simulink model "six_plus_six_AcmsteeringV09_main_2lflm"  (R2014a)
settings: Solver=FixedStepDiscrete  StartTime=0.0  StopTime=10.0  FixedStep=0.0005  RelTol=1e-3
InitFcn:
  | Veh_Par_wxt
undefined symbols (not defined in the file or in its folder): acc_spdctl, ag_thr, B, bra_em, bra_pre_gz2, bra_pre_gz34, bra_pre_yd, brakepre_dem_data, brakeTrq_dem_data, bratrq_max, ecucoder_acal, eff_tran, ESP_switch, G, guzhang_lf, guzhang_lm, guzhang_lr, guzhang_rf, guzhang_rm, guzhang_rr, kd1, kd2, ki1, ki2, kp1, kp2, L, myFIS, premax, Radius, RC_switch, s_opt_yi, s_opt_zhuan, s_opt_zhuan_add, s_opt_zhuan_table, spd_map_mot, spd_spdctl, speed_thr_park, TCS_switch, tras_ratio, trq_map_mot, trqmax_yd, trqmax_zx, trqmaxneg, v_gain, v_table, v_thr_park, zhidong_bianmazhi, zhidong_down, zhidong_up, zhidong_youmen, zhuanxiang_bianmazhi, zhuanxiang_down, zhuanxiang_up, zhuanxiang_youmen
libraries: simulink x980, ec5744lib x59, fuzblock x2
(part 6 of 25)

== system six_plus_six_AcmsteeringV09_main_2lflm/Data_input/BMS4_2/BMS4 ==
  input : Inport
  Enable : EnablePort
  BMS4_InputVolACC_Ad : Sum
  BMS4_InputVolACC_Convert : DataTypeConversion  OutDataTypeStr=uint32
  BMS4_InputVolACC_F : Gain  Gain=0.1
  BMS4_InputVolACC_L : simulink/Logic and Bit Operations/Bitwise Operator  logicop=AND  UseBitMask=on  BitMask=65535  BitMaskRealWorld=Stored Integer
  BMS4_InputVolACC_O : Constant  Value=0  OutDataTypeStr=single
  BMS4_InputVolACC_S : ArithShift
  BMS4_InputVolACC_Sub : Subsystem
  BMS4_InputVolACC_sat : Saturate  UpperLimit=6553.5  LowerLimit=0
  BMS4_InputVolACCcv : DataTypeConversion
  BMS4_InputVolACCinput2_Ad : Sum
  BMS4_InputVolACCinput2_C : Constant  Value=256
  BMS4_InputVolACCinput2_P : Product
  BMS4_InputVolCHG_Ad : Sum
  BMS4_InputVolCHG_Convert : DataTypeConversion  OutDataTypeStr=uint32
  BMS4_InputVolCHG_F : Gain  Gain=0.1
  BMS4_InputVolCHG_L : simulink/Logic and Bit Operations/Bitwise Operator  logicop=AND  UseBitMask=on  BitMask=65535  BitMaskRealWorld=Stored Integer
  BMS4_InputVolCHG_O : Constant  Value=0  OutDataTypeStr=single
  BMS4_InputVolCHG_S : ArithShift
  BMS4_InputVolCHG_Sub : Subsystem
  BMS4_InputVolCHG_sat : Saturate  UpperLimit=6553.5  LowerLimit=0
  BMS4_InputVolCHGcv : DataTypeConversion
  BMS4_InputVolCHGinput6_Ad : Sum
  BMS4_InputVolCHGinput6_C : Constant  Value=256
  BMS4_InputVolCHGinput6_P : Product
  BMS4_InputVolKEYON_Ad : Sum
  BMS4_InputVolKEYON_Convert : DataTypeConversion  OutDataTypeStr=uint32
  BMS4_InputVolKEYON_F : Gain  Gain=0.1
  BMS4_InputVolKEYON_L : simulink/Logic and Bit Operations/Bitwise Operator  logicop=AND  UseBitMask=on  BitMask=65535  BitMaskRealWorld=Stored Integer
  BMS4_InputVolKEYON_O : Constant  Value=0  OutDataTypeStr=single
  BMS4_InputVolKEYON_S : ArithShift
  BMS4_InputVolKEYON_Sub : Subsystem
  BMS4_InputVolKEYON_sat : Saturate  UpperLimit=6553.5  LowerLimit=0
  BMS4_InputVolKEYONcv : DataTypeConversion
  BMS4_InputVolKEYONinput4_Ad : Sum
  BMS4_InputVolKEYONinput4_C : Constant  Value=256
  BMS4_InputVolKEYONinput4_P : Product
  BMS4_Sys_Status3_Ad : Sum
  BMS4_Sys_Status3_Convert : DataTypeConversion  OutDataTypeStr=uint32
  BMS4_Sys_Status3_F : Gain
  BMS4_Sys_Status3_L : simulink/Logic and Bit Operations/Bitwise Operator  logicop=AND  UseBitMask=on  BitMask=255  BitMaskRealWorld=Stored Integer
  BMS4_Sys_Status3_O : Constant  Value=0  OutDataTypeStr=single
  BMS4_Sys_Status3_S : ArithShift
  BMS4_Sys_Status3_Sub : Subsystem
  BMS4_Sys_Status3_sat : Saturate  UpperLimit=255  LowerLimit=0
  BMS4_Sys_Status3cv : DataTypeConversion
  Demux : Demux  Outputs=8
  BMS4_Sys_Status3_Out : Outport
  BMS4_InputVolKEYON_Out : Outport  Port=2
  BMS4_InputVolCHG_Out : Outport  Port=3
  BMS4_InputVolACC_Out : Outport  Port=4
  wires:
  BMS4_Sys_Status3_F/1 -> BMS4_Sys_Status3_Ad/1
  BMS4_Sys_Status3_O/1 -> BMS4_Sys_Status3_Ad/2
  BMS4_Sys_Status3_Ad/1 -> BMS4_Sys_Status3_sat/1
  BMS4_Sys_Status3_sat/1 -> BMS4_Sys_Status3_Out/1
  Demux/1 -> BMS4_Sys_Status3_Sub/1(In1)
  BMS4_Sys_Status3_Sub/1(Out1) -> BMS4_Sys_Status3_Convert/1
  BMS4_Sys_Status3_Convert/1 -> BMS4_Sys_Status3_L/1
  BMS4_Sys_Status3_L/1 -> BMS4_Sys_Status3_S/1
  BMS4_Sys_Status3_S/1 -> BMS4_Sys_Status3cv/1
  BMS4_Sys_Status3cv/1 -> BMS4_Sys_Status3_F/1
  BMS4_InputVolKEYON_F/1 -> BMS4_InputVolKEYON_Ad/1
  BMS4_InputVolKEYON_O/1 -> BMS4_InputVolKEYON_Ad/2
  BMS4_InputVolKEYON_Ad/1 -> BMS4_InputVolKEYON_sat/1
  BMS4_InputVolKEYON_sat/1 -> BMS4_InputVolKEYON_Out/1
  Demux/4 -> BMS4_InputVolKEYONinput4_P/1
  BMS4_InputVolKEYONinput4_C/1 -> BMS4_InputVolKEYONinput4_P/2
  BMS4_InputVolKEYONinput4_P/1 -> BMS4_InputVolKEYONinput4_Ad/1
  Demux/5 -> BMS4_InputVolKEYONinput4_Ad/2
  BMS4_InputVolKEYONinput4_Ad/1 -> BMS4_InputVolKEYON_Sub/1(In1)
  BMS4_InputVolKEYON_Sub/1(Out1) -> BMS4_InputVolKEYON_Convert/1
  BMS4_InputVolKEYON_Convert/1 -> BMS4_InputVolKEYON_L/1
  BMS4_InputVolKEYON_L/1 -> BMS4_InputVolKEYON_S/1
  BMS4_InputVolKEYON_S/1 -> BMS4_InputVolKEYONcv/1
  BMS4_InputVolKEYONcv/1 -> BMS4_InputVolKEYON_F/1
  BMS4_InputVolCHG_F/1 -> BMS4_InputVolCHG_Ad/1
  BMS4_InputVolCHG_O/1 -> BMS4_InputVolCHG_Ad/2
  BMS4_InputVolCHG_Ad/1 -> BMS4_InputVolCHG_sat/1
  BMS4_InputVolCHG_sat/1 -> BMS4_InputVolCHG_Out/1
  Demux/6 -> BMS4_InputVolCHGinput6_P/1
  BMS4_InputVolCHGinput6_C/1 -> BMS4_InputVolCHGinput6_P/2
  BMS4_InputVolCHGinput6_P/1 -> BMS4_InputVolCHGinput6_Ad/1
  Demux/7 -> BMS4_InputVolCHGinput6_Ad/2
  BMS4_InputVolCHGinput6_Ad/1 -> BMS4_InputVolCHG_Sub/1(In1)
  BMS4_InputVolCHG_Sub/1(Out1) -> BMS4_InputVolCHG_Convert/1
  BMS4_InputVolCHG_Convert/1 -> BMS4_InputVolCHG_L/1
  BMS4_InputVolCHG_L/1 -> BMS4_InputVolCHG_S/1
  BMS4_InputVolCHG_S/1 -> BMS4_InputVolCHGcv/1
  BMS4_InputVolCHGcv/1 -> BMS4_InputVolCHG_F/1
  BMS4_InputVolACC_F/1 -> BMS4_InputVolACC_Ad/1
  BMS4_InputVolACC_O/1 -> BMS4_InputVolACC_Ad/2
  BMS4_InputVolACC_Ad/1 -> BMS4_InputVolACC_sat/1
  BMS4_InputVolACC_sat/1 -> BMS4_InputVolACC_Out/1
  Demux/2 -> BMS4_InputVolACCinput2_P/1
  BMS4_InputVolACCinput2_C/1 -> BMS4_InputVolACCinput2_P/2
  BMS4_InputVolACCinput2_P/1 -> BMS4_InputVolACCinput2_Ad/1
  Demux/3 -> BMS4_InputVolACCinput2_Ad/2
  BMS4_InputVolACCinput2_Ad/1 -> BMS4_InputVolACC_Sub/1(In1)
  BMS4_InputVolACC_Sub/1(Out1) -> BMS4_InputVolACC_Convert/1
  BMS4_InputVolACC_Convert/1 -> BMS4_InputVolACC_L/1
  BMS4_InputVolACC_L/1 -> BMS4_InputVolACC_S/1
  BMS4_InputVolACC_S/1 -> BMS4_InputVolACCcv/1
  BMS4_InputVolACCcv/1 -> BMS4_InputVolACC_F/1
  input/1 -> Demux/1

== system six_plus_six_AcmsteeringV09_main_2lflm/Data_input/BMS5/BMS5 ==
  input : Inport
  Enable : EnablePort
  BMS5_15s_InstanceDisPower_Ad : Sum
  BMS5_15s_InstanceDisPower_Convert : DataTypeConversion  OutDataTypeStr=uint32
  BMS5_15s_InstanceDisPower_F : Gain  Gain=0.01
  BMS5_15s_InstanceDisPower_L : simulink/Logic and Bit Operations/Bitwise Operator  logicop=AND  UseBitMask=on  BitMask=65535  BitMaskRealWorld=Stored Integer
  BMS5_15s_InstanceDisPower_O : Constant  Value=0  OutDataTypeStr=single
  BMS5_15s_InstanceDisPower_S : ArithShift
  BMS5_15s_InstanceDisPower_Sub : Subsystem
  BMS5_15s_InstanceDisPower_sat : Saturate  UpperLimit=655.35  LowerLimit=0
  BMS5_15s_InstanceDisPowercv : DataTypeConversion
  BMS5_15s_InstanceDisPowerinput4_Ad : Sum
  BMS5_15s_InstanceDisPowerinput4_C : Constant  Value=256
  BMS5_15s_InstanceDisPowerinput4_P : Product
  BMS5_ContDischargePower_Ad : Sum
  BMS5_ContDischargePower_Convert : DataTypeConversion  OutDataTypeStr=uint32
  BMS5_ContDischargePower_F : Gain  Gain=0.01
  BMS5_ContDischargePower_L : simulink/Logic and Bit Operations/Bitwise Operator  logicop=AND  UseBitMask=on  BitMask=65535  BitMaskRealWorld=Stored Integer
  BMS5_ContDischargePower_O : Constant  Value=0  OutDataTypeStr=single
  BMS5_ContDischargePower_S : ArithShift
  BMS5_ContDischargePower_Sub : Subsystem
  BMS5_ContDischargePower_sat : Saturate  UpperLimit=655.35  LowerLimit=0
  BMS5_ContDischargePowercv : DataTypeConversion
  BMS5_ContDischargePowerinput2_Ad : Sum
  BMS5_ContDischargePowerinput2_C : Constant  Value=256
  BMS5_ContDischargePowerinput2_P : Product
  BMS5_FailureLevel_Ad : Sum
  BMS5_FailureLevel_Convert : DataTypeConversion  OutDataTypeStr=uint32
  BMS5_FailureLevel_F : Gain
  BMS5_FailureLevel_L : simulink/Logic and Bit Operations/Bitwise Operator  logicop=AND  UseBitMask=on  BitMask=255  BitMaskRealWorld=Stored Integer
  BMS5_FailureLevel_O : Constant  Value=0  OutDataTypeStr=single
  BMS5_FailureLevel_S : ArithShift
  BMS5_FailureLevel_Sub : Subsystem
  BMS5_FailureLevel_sat : Saturate  UpperLimit=255  LowerLimit=0
  BMS5_FailureLevelcv : DataTypeConversion
  BMS5_FeedbackPower_Ad : Sum
  BMS5_FeedbackPower_Convert : DataTypeConversion  OutDataTypeStr=uint32
  BMS5_FeedbackPower_F : Gain  Gain=0.01
  BMS5_FeedbackPower_L : simulink/Logic and Bit Operations/Bitwise Operator  logicop=AND  UseBitMask=on  BitMask=65535  BitMaskRealWorld=Stored Integer
  BMS5_FeedbackPower_O : Constant  Value=0  OutDataTypeStr=single
  BMS5_FeedbackPower_S : ArithShift
  BMS5_FeedbackPower_Sub : Subsystem
  BMS5_FeedbackPower_sat : Saturate  UpperLimit=655.35  LowerLimit=0
  BMS5_FeedbackPowercv : DataTypeConversion
  BMS5_FeedbackPowerinput6_Ad : Sum
  BMS5_FeedbackPowerinput6_C : Constant  Value=256
  BMS5_FeedbackPowerinput6_P : Product
  BMS5_UpDownRequest_Ad : Sum
  BMS5_UpDownRequest_Convert : DataTypeConversion  OutDataTypeStr=uint32
  BMS5_UpDownRequest_F : Gain
  BMS5_UpDownRequest_L : simulink/Logic and Bit Operations/Bitwise Operator  logicop=AND  UseBitMask=on  BitMask=255  BitMaskRealWorld=Stored Integer
  BMS5_UpDownRequest_O : Constant  Value=0  OutDataTypeStr=single
  BMS5_UpDownRequest_S : ArithShift
  BMS5_UpDownRequest_Sub : Subsystem
  BMS5_UpDownRequest_sat : Saturate  UpperLimit=255  LowerLimit=0
  BMS5_UpDownRequestcv : DataTypeConversion
  Demux : Demux  Outputs=8
  BMS5_UpDownRequest_Out : Outport
  BMS5_FeedbackPower_Out : Outport  Port=2
  BMS5_FailureLevel_Out : Outport  Port=3
  BMS5_ContDischargePower_Out : Outport  Port=4
  BMS5_15s_InstanceDisPower_Out : Outport  Port=5
  wires:
  BMS5_UpDownRequest_F/1 -> BMS5_UpDownRequest_Ad/1
  BMS5_UpDownRequest_O/1 -> BMS5_UpDownRequest_Ad/2
  BMS5_UpDownRequest_Ad/1 -> BMS5_UpDownRequest_sat/1
  BMS5_UpDownRequest_sat/1 -> BMS5_UpDownRequest_Out/1
  Demux/8 -> BMS5_UpDownRequest_Sub/1(In1)
  BMS5_UpDownRequest_Sub/1(Out1) -> BMS5_UpDownRequest_Convert/1
  BMS5_UpDownRequest_Convert/1 -> BMS5_UpDownRequest_L/1
  BMS5_UpDownRequest_L/1 -> BMS5_UpDownRequest_S/1
  BMS5_UpDownRequest_S/1 -> BMS5_UpDownRequestcv/1
  BMS5_UpDownRequestcv/1 -> BMS5_UpDownRequest_F/1
  BMS5_FeedbackPower_F/1 -> BMS5_FeedbackPower_Ad/1
  BMS5_FeedbackPower_O/1 -> BMS5_FeedbackPower_Ad/2
  BMS5_FeedbackPower_Ad/1 -> BMS5_FeedbackPower_sat/1
  BMS5_FeedbackPower_sat/1 -> BMS5_FeedbackPower_Out/1
  Demux/6 -> BMS5_FeedbackPowerinput6_P/1
  BMS5_FeedbackPowerinput6_C/1 -> BMS5_FeedbackPowerinput6_P/2
  BMS5_FeedbackPowerinput6_P/1 -> BMS5_FeedbackPowerinput6_Ad/1
  Demux/7 -> BMS5_FeedbackPowerinput6_Ad/2
  BMS5_FeedbackPowerinput6_Ad/1 -> BMS5_FeedbackPower_Sub/1(In1)
  BMS5_FeedbackPower_Sub/1(Out1) -> BMS5_FeedbackPower_Convert/1
  BMS5_FeedbackPower_Convert/1 -> BMS5_FeedbackPower_L/1
  BMS5_FeedbackPower_L/1 -> BMS5_FeedbackPower_S/1
  BMS5_FeedbackPower_S/1 -> BMS5_FeedbackPowercv/1
  BMS5_FeedbackPowercv/1 -> BMS5_FeedbackPower_F/1
  BMS5_FailureLevel_F/1 -> BMS5_FailureLevel_Ad/1
  BMS5_FailureLevel_O/1 -> BMS5_FailureLevel_Ad/2
  BMS5_FailureLevel_Ad/1 -> BMS5_FailureLevel_sat/1
  BMS5_FailureLevel_sat/1 -> BMS5_FailureLevel_Out/1
  Demux/1 -> BMS5_FailureLevel_Sub/1(In1)
  BMS5_FailureLevel_Sub/1(Out1) -> BMS5_FailureLevel_Convert/1
  BMS5_FailureLevel_Convert/1 -> BMS5_FailureLevel_L/1
  BMS5_FailureLevel_L/1 -> BMS5_FailureLevel_S/1
  BMS5_FailureLevel_S/1 -> BMS5_FailureLevelcv/1
  BMS5_FailureLevelcv/1 -> BMS5_FailureLevel_F/1
  BMS5_ContDischargePower_F/1 -> BMS5_ContDischargePower_Ad/1
  BMS5_ContDischargePower_O/1 -> BMS5_ContDischargePower_Ad/2
  BMS5_ContDischargePower_Ad/1 -> BMS5_ContDischargePower_sat/1
  BMS5_ContDischargePower_sat/1 -> BMS5_ContDischargePower_Out/1
  Demux/2 -> BMS5_ContDischargePowerinput2_P/1
  BMS5_ContDischargePowerinput2_C/1 -> BMS5_ContDischargePowerinput2_P/2
  BMS5_ContDischargePowerinput2_P/1 -> BMS5_ContDischargePowerinput2_Ad/1
  Demux/3 -> BMS5_ContDischargePowerinput2_Ad/2
  BMS5_ContDischargePowerinput2_Ad/1 -> BMS5_ContDischargePower_Sub/1(In1)
  BMS5_ContDischargePower_Sub/1(Out1) -> BMS5_ContDischargePower_Convert/1
  BMS5_ContDischargePower_Convert/1 -> BMS5_ContDischargePower_L/1
  BMS5_ContDischargePower_L/1 -> BMS5_ContDischargePower_S/1
  BMS5_ContDischargePower_S/1 -> BMS5_ContDischargePowercv/1
  BMS5_ContDischargePowercv/1 -> BMS5_ContDischargePower_F/1
  BMS5_15s_InstanceDisPower_F/1 -> BMS5_15s_InstanceDisPower_Ad/1
  BMS5_15s_InstanceDisPower_O/1 -> BMS5_15s_InstanceDisPower_Ad/2
  BMS5_15s_InstanceDisPower_Ad/1 -> BMS5_15s_InstanceDisPower_sat/1
  BMS5_15s_InstanceDisPower_sat/1 -> BMS5_15s_InstanceDisPower_Out/1
  Demux/4 -> BMS5_15s_InstanceDisPowerinput4_P/1
  BMS5_15s_InstanceDisPowerinput4_C/1 -> BMS5_15s_InstanceDisPowerinput4_P/2
  BMS5_15s_InstanceDisPowerinput4_P/1 -> BMS5_15s_InstanceDisPowerinput4_Ad/1
  Demux/5 -> BMS5_15s_InstanceDisPowerinput4_Ad/2
  BMS5_15s_InstanceDisPowerinput4_Ad/1 -> BMS5_15s_InstanceDisPower_Sub/1(In1)
  BMS5_15s_InstanceDisPower_Sub/1(Out1) -> BMS5_15s_InstanceDisPower_Convert/1
  BMS5_15s_InstanceDisPower_Convert/1 -> BMS5_15s_InstanceDisPower_L/1
  BMS5_15s_InstanceDisPower_L/1 -> BMS5_15s_InstanceDisPower_S/1
  BMS5_15s_InstanceDisPower_S/1 -> BMS5_15s_InstanceDisPowercv/1
  BMS5_15s_InstanceDisPowercv/1 -> BMS5_15s_InstanceDisPower_F/1
  input/1 -> Demux/1

== system six_plus_six_AcmsteeringV09_main_2lflm/Data_input/BMS5_1/BMS5 ==
  input : Inport
  Enable : EnablePort
  BMS5_15s_InstanceDisPower_Ad : Sum
  BMS5_15s_InstanceDisPower_Convert : DataTypeConversion  OutDataTypeStr=uint32
  BMS5_15s_InstanceDisPower_F : Gain  Gain=0.01
  BMS5_15s_InstanceDisPower_L : simulink/Logic and Bit Operations/Bitwise Operator  logicop=AND  UseBitMask=on  BitMask=65535  BitMaskRealWorld=Stored Integer
  BMS5_15s_InstanceDisPower_O : Constant  Value=0  OutDataTypeStr=single
  BMS5_15s_InstanceDisPower_S : ArithShift
  BMS5_15s_InstanceDisPower_Sub : Subsystem
  BMS5_15s_InstanceDisPower_sat : Saturate  UpperLimit=655.35  LowerLimit=0
  BMS5_15s_InstanceDisPowercv : DataTypeConversion
  BMS5_15s_InstanceDisPowerinput4_Ad : Sum
  BMS5_15s_InstanceDisPowerinput4_C : Constant  Value=256
  BMS5_15s_InstanceDisPowerinput4_P : Product
  BMS5_ContDischargePower_Ad : Sum
  BMS5_ContDischargePower_Convert : DataTypeConversion  OutDataTypeStr=uint32
  BMS5_ContDischargePower_F : Gain  Gain=0.01
  BMS5_ContDischargePower_L : simulink/Logic and Bit Operations/Bitwise Operator  logicop=AND  UseBitMask=on  BitMask=65535  BitMaskRealWorld=Stored Integer
  BMS5_ContDischargePower_O : Constant  Value=0  OutDataTypeStr=single
  BMS5_ContDischargePower_S : ArithShift
  BMS5_ContDischargePower_Sub : Subsystem
  BMS5_ContDischargePower_sat : Saturate  UpperLimit=655.35  LowerLimit=0
  BMS5_ContDischargePowercv : DataTypeConversion
  BMS5_ContDischargePowerinput2_Ad : Sum
  BMS5_ContDischargePowerinput2_C : Constant  Value=256
  BMS5_ContDischargePowerinput2_P : Product
  BMS5_FailureLevel_Ad : Sum
  BMS5_FailureLevel_Convert : DataTypeConversion  OutDataTypeStr=uint32
  BMS5_FailureLevel_F : Gain
  BMS5_FailureLevel_L : simulink/Logic and Bit Operations/Bitwise Operator  logicop=AND  UseBitMask=on  BitMask=255  BitMaskRealWorld=Stored Integer
  BMS5_FailureLevel_O : Constant  Value=0  OutDataTypeStr=single
  BMS5_FailureLevel_S : ArithShift
  BMS5_FailureLevel_Sub : Subsystem
  BMS5_FailureLevel_sat : Saturate  UpperLimit=255  LowerLimit=0
  BMS5_FailureLevelcv : DataTypeConversion
  BMS5_FeedbackPower_Ad : Sum
  BMS5_FeedbackPower_Convert : DataTypeConversion  OutDataTypeStr=uint32
  BMS5_FeedbackPower_F : Gain  Gain=0.01
  BMS5_FeedbackPower_L : simulink/Logic and Bit Operations/Bitwise Operator  logicop=AND  UseBitMask=on  BitMask=65535  BitMaskRealWorld=Stored Integer
  BMS5_FeedbackPower_O : Constant  Value=0  OutDataTypeStr=single
  BMS5_FeedbackPower_S : ArithShift
  BMS5_FeedbackPower_Sub : Subsystem
  BMS5_FeedbackPower_sat : Saturate  UpperLimit=655.35  LowerLimit=0
  BMS5_FeedbackPowercv : DataTypeConversion
  BMS5_FeedbackPowerinput6_Ad : Sum
  BMS5_FeedbackPowerinput6_C : Constant  Value=256
  BMS5_FeedbackPowerinput6_P : Product
  BMS5_UpDownRequest_Ad : Sum
  BMS5_UpDownRequest_Convert : DataTypeConversion  OutDataTypeStr=uint32
  BMS5_UpDownRequest_F : Gain
  BMS5_UpDownRequest_L : simulink/Logic and Bit Operations/Bitwise Operator  logicop=AND  UseBitMask=on  BitMask=255  BitMaskRealWorld=Stored Integer
  BMS5_UpDownRequest_O : Constant  Value=0  OutDataTypeStr=single
  BMS5_UpDownRequest_S : ArithShift
  BMS5_UpDownRequest_Sub : Subsystem
  BMS5_UpDownRequest_sat : Saturate  UpperLimit=255  LowerLimit=0
  BMS5_UpDownRequestcv : DataTypeConversion
  Demux : Demux  Outputs=8
  BMS5_UpDownRequest_Out : Outport
  BMS5_FeedbackPower_Out : Outport  Port=2
  BMS5_FailureLevel_Out : Outport  Port=3
  BMS5_ContDischargePower_Out : Outport  Port=4
  BMS5_15s_InstanceDisPower_Out : Outport  Port=5
  wires:
  BMS5_UpDownRequest_F/1 -> BMS5_UpDownRequest_Ad/1
  BMS5_UpDownRequest_O/1 -> BMS5_UpDownRequest_Ad/2
  BMS5_UpDownRequest_Ad/1 -> BMS5_UpDownRequest_sat/1
  BMS5_UpDownRequest_sat/1 -> BMS5_UpDownRequest_Out/1
  Demux/8 -> BMS5_UpDownRequest_Sub/1(In1)
  BMS5_UpDownRequest_Sub/1(Out1) -> BMS5_UpDownRequest_Convert/1
  BMS5_UpDownRequest_Convert/1 -> BMS5_UpDownRequest_L/1
  BMS5_UpDownRequest_L/1 -> BMS5_UpDownRequest_S/1
  BMS5_UpDownRequest_S/1 -> BMS5_UpDownRequestcv/1
  BMS5_UpDownRequestcv/1 -> BMS5_UpDownRequest_F/1
  BMS5_FeedbackPower_F/1 -> BMS5_FeedbackPower_Ad/1
  BMS5_FeedbackPower_O/1 -> BMS5_FeedbackPower_Ad/2
  BMS5_FeedbackPower_Ad/1 -> BMS5_FeedbackPower_sat/1
  BMS5_FeedbackPower_sat/1 -> BMS5_FeedbackPower_Out/1
  Demux/6 -> BMS5_FeedbackPowerinput6_P/1
  BMS5_FeedbackPowerinput6_C/1 -> BMS5_FeedbackPowerinput6_P/2
  BMS5_FeedbackPowerinput6_P/1 -> BMS5_FeedbackPowerinput6_Ad/1
  Demux/7 -> BMS5_FeedbackPowerinput6_Ad/2
  BMS5_FeedbackPowerinput6_Ad/1 -> BMS5_FeedbackPower_Sub/1(In1)
  BMS5_FeedbackPower_Sub/1(Out1) -> BMS5_FeedbackPower_Convert/1
  BMS5_FeedbackPower_Convert/1 -> BMS5_FeedbackPower_L/1
  BMS5_FeedbackPower_L/1 -> BMS5_FeedbackPower_S/1
  BMS5_FeedbackPower_S/1 -> BMS5_FeedbackPowercv/1
  BMS5_FeedbackPowercv/1 -> BMS5_FeedbackPower_F/1
  BMS5_FailureLevel_F/1 -> BMS5_FailureLevel_Ad/1
  BMS5_FailureLevel_O/1 -> BMS5_FailureLevel_Ad/2
  BMS5_FailureLevel_Ad/1 -> BMS5_FailureLevel_sat/1
  BMS5_FailureLevel_sat/1 -> BMS5_FailureLevel_Out/1
  Demux/1 -> BMS5_FailureLevel_Sub/1(In1)
  BMS5_FailureLevel_Sub/1(Out1) -> BMS5_FailureLevel_Convert/1
  BMS5_FailureLevel_Convert/1 -> BMS5_FailureLevel_L/1
  BMS5_FailureLevel_L/1 -> BMS5_FailureLevel_S/1
  BMS5_FailureLevel_S/1 -> BMS5_FailureLevelcv/1
  BMS5_FailureLevelcv/1 -> BMS5_FailureLevel_F/1
  BMS5_ContDischargePower_F/1 -> BMS5_ContDischargePower_Ad/1
  BMS5_ContDischargePower_O/1 -> BMS5_ContDischargePower_Ad/2
  BMS5_ContDischargePower_Ad/1 -> BMS5_ContDischargePower_sat/1
  BMS5_ContDischargePower_sat/1 -> BMS5_ContDischargePower_Out/1
  Demux/2 -> BMS5_ContDischargePowerinput2_P/1
  BMS5_ContDischargePowerinput2_C/1 -> BMS5_ContDischargePowerinput2_P/2
  BMS5_ContDischargePowerinput2_P/1 -> BMS5_ContDischargePowerinput2_Ad/1
  Demux/3 -> BMS5_ContDischargePowerinput2_Ad/2
  BMS5_ContDischargePowerinput2_Ad/1 -> BMS5_ContDischargePower_Sub/1(In1)
  BMS5_ContDischargePower_Sub/1(Out1) -> BMS5_ContDischargePower_Convert/1
  BMS5_ContDischargePower_Convert/1 -> BMS5_ContDischargePower_L/1
  BMS5_ContDischargePower_L/1 -> BMS5_ContDischargePower_S/1
  BMS5_ContDischargePower_S/1 -> BMS5_ContDischargePowercv/1
  BMS5_ContDischargePowercv/1 -> BMS5_ContDischargePower_F/1
  BMS5_15s_InstanceDisPower_F/1 -> BMS5_15s_InstanceDisPower_Ad/1
  BMS5_15s_InstanceDisPower_O/1 -> BMS5_15s_InstanceDisPower_Ad/2
  BMS5_15s_InstanceDisPower_Ad/1 -> BMS5_15s_InstanceDisPower_sat/1
  BMS5_15s_InstanceDisPower_sat/1 -> BMS5_15s_InstanceDisPower_Out/1
  Demux/4 -> BMS5_15s_InstanceDisPowerinput4_P/1
  BMS5_15s_InstanceDisPowerinput4_C/1 -> BMS5_15s_InstanceDisPowerinput4_P/2
  BMS5_15s_InstanceDisPowerinput4_P/1 -> BMS5_15s_InstanceDisPowerinput4_Ad/1
  Demux/5 -> BMS5_15s_InstanceDisPowerinput4_Ad/2
  BMS5_15s_InstanceDisPowerinput4_Ad/1 -> BMS5_15s_InstanceDisPower_Sub/1(In1)
  BMS5_15s_InstanceDisPower_Sub/1(Out1) -> BMS5_15s_InstanceDisPower_Convert/1
  BMS5_15s_InstanceDisPower_Convert/1 -> BMS5_15s_InstanceDisPower_L/1
  BMS5_15s_InstanceDisPower_L/1 -> BMS5_15s_InstanceDisPower_S/1
  BMS5_15s_InstanceDisPower_S/1 -> BMS5_15s_InstanceDisPowercv/1
  BMS5_15s_InstanceDisPowercv/1 -> BMS5_15s_InstanceDisPower_F/1
  input/1 -> Demux/1

== system six_plus_six_AcmsteeringV09_main_2lflm/Data_input/BMS5_2/BMS5 ==
  input : Inport
  Enable : EnablePort
  BMS5_15s_InstanceDisPower_Ad : Sum
  BMS5_15s_InstanceDisPower_Convert : DataTypeConversion  OutDataTypeStr=uint32
  BMS5_15s_InstanceDisPower_F : Gain  Gain=0.01
  BMS5_15s_InstanceDisPower_L : simulink/Logic and Bit Operations/Bitwise Operator  logicop=AND  UseBitMask=on  BitMask=65535  BitMaskRealWorld=Stored Integer
  BMS5_15s_InstanceDisPower_O : Constant  Value=0  OutDataTypeStr=single
  BMS5_15s_InstanceDisPower_S : ArithShift
  BMS5_15s_InstanceDisPower_Sub : Subsystem
  BMS5_15s_InstanceDisPower_sat : Saturate  UpperLimit=655.35  LowerLimit=0
  BMS5_15s_InstanceDisPowercv : DataTypeConversion
  BMS5_15s_InstanceDisPowerinput4_Ad : Sum
  BMS5_15s_InstanceDisPowerinput4_C : Constant  Value=256
  BMS5_15s_InstanceDisPowerinput4_P : Product
  BMS5_ContDischargePower_Ad : Sum
  BMS5_ContDischargePower_Convert : DataTypeConversion  OutDataTypeStr=uint32
  BMS5_ContDischargePower_F : Gain  Gain=0.01
  BMS5_ContDischargePower_L : simulink/Logic and Bit Operations/Bitwise Operator  logicop=AND  UseBitMask=on  BitMask=65535  BitMaskRealWorld=Stored Integer
  BMS5_ContDischargePower_O : Constant  Value=0  OutDataTypeStr=single
  BMS5_ContDischargePower_S : ArithShift
  BMS5_ContDischargePower_Sub : Subsystem
  BMS5_ContDischargePower_sat : Saturate  UpperLimit=655.35  LowerLimit=0
  BMS5_ContDischargePowercv : DataTypeConversion
  BMS5_ContDischargePowerinput2_Ad : Sum
  BMS5_ContDischargePowerinput2_C : Constant  Value=256
  BMS5_ContDischargePowerinput2_P : Product
  BMS5_FailureLevel_Ad : Sum
  BMS5_FailureLevel_Convert : DataTypeConversion  OutDataTypeStr=uint32
  BMS5_FailureLevel_F : Gain
  BMS5_FailureLevel_L : simulink/Logic and Bit Operations/Bitwise Operator  logicop=AND  UseBitMask=on  BitMask=255  BitMaskRealWorld=Stored Integer
  BMS5_FailureLevel_O : Constant  Value=0  OutDataTypeStr=single
  BMS5_FailureLevel_S : ArithShift
  BMS5_FailureLevel_Sub : Subsystem
  BMS5_FailureLevel_sat : Saturate  UpperLimit=255  LowerLimit=0
  BMS5_FailureLevelcv : DataTypeConversion
  BMS5_FeedbackPower_Ad : Sum
  BMS5_FeedbackPower_Convert : DataTypeConversion  OutDataTypeStr=uint32
  BMS5_FeedbackPower_F : Gain  Gain=0.01
  BMS5_FeedbackPower_L : simulink/Logic and Bit Operations/Bitwise Operator  logicop=AND  UseBitMask=on  BitMask=65535  BitMaskRealWorld=Stored Integer
  BMS5_FeedbackPower_O : Constant  Value=0  OutDataTypeStr=single
  BMS5_FeedbackPower_S : ArithShift
  BMS5_FeedbackPower_Sub : Subsystem
  BMS5_FeedbackPower_sat : Saturate  UpperLimit=655.35  LowerLimit=0
  BMS5_FeedbackPowercv : DataTypeConversion
  BMS5_FeedbackPowerinput6_Ad : Sum
  BMS5_FeedbackPowerinput6_C : Constant  Value=256
  BMS5_FeedbackPowerinput6_P : Product
  BMS5_UpDownRequest_Ad : Sum
  BMS5_UpDownRequest_Convert : DataTypeConversion  OutDataTypeStr=uint32
  BMS5_UpDownRequest_F : Gain
  BMS5_UpDownRequest_L : simulink/Logic and Bit Operations/Bitwise Operator  logicop=AND  UseBitMask=on  BitMask=255  BitMaskRealWorld=Stored Integer
  BMS5_UpDownRequest_O : Constant  Value=0  OutDataTypeStr=single
  BMS5_UpDownRequest_S : ArithShift
  BMS5_UpDownRequest_Sub : Subsystem
  BMS5_UpDownRequest_sat : Saturate  UpperLimit=255  LowerLimit=0
  BMS5_UpDownRequestcv : DataTypeConversion
  Demux : Demux  Outputs=8
  BMS5_UpDownRequest_Out : Outport
  BMS5_FeedbackPower_Out : Outport  Port=2
  BMS5_FailureLevel_Out : Outport  Port=3
  BMS5_ContDischargePower_Out : Outport  Port=4
  BMS5_15s_InstanceDisPower_Out : Outport  Port=5
  wires:
  BMS5_UpDownRequest_F/1 -> BMS5_UpDownRequest_Ad/1
  BMS5_UpDownRequest_O/1 -> BMS5_UpDownRequest_Ad/2
  BMS5_UpDownRequest_Ad/1 -> BMS5_UpDownRequest_sat/1
  BMS5_UpDownRequest_sat/1 -> BMS5_UpDownRequest_Out/1
  Demux/8 -> BMS5_UpDownRequest_Sub/1(In1)
  BMS5_UpDownRequest_Sub/1(Out1) -> BMS5_UpDownRequest_Convert/1
  BMS5_UpDownRequest_Convert/1 -> BMS5_UpDownRequest_L/1
  BMS5_UpDownRequest_L/1 -> BMS5_UpDownRequest_S/1
  BMS5_UpDownRequest_S/1 -> BMS5_UpDownRequestcv/1
  BMS5_UpDownRequestcv/1 -> BMS5_UpDownRequest_F/1
  BMS5_FeedbackPower_F/1 -> BMS5_FeedbackPower_Ad/1
  BMS5_FeedbackPower_O/1 -> BMS5_FeedbackPower_Ad/2
  BMS5_FeedbackPower_Ad/1 -> BMS5_FeedbackPower_sat/1
  BMS5_FeedbackPower_sat/1 -> BMS5_FeedbackPower_Out/1
  Demux/6 -> BMS5_FeedbackPowerinput6_P/1
  BMS5_FeedbackPowerinput6_C/1 -> BMS5_FeedbackPowerinput6_P/2
  BMS5_FeedbackPowerinput6_P/1 -> BMS5_FeedbackPowerinput6_Ad/1
  Demux/7 -> BMS5_FeedbackPowerinput6_Ad/2
  BMS5_FeedbackPowerinput6_Ad/1 -> BMS5_FeedbackPower_Sub/1(In1)
  BMS5_FeedbackPower_Sub/1(Out1) -> BMS5_FeedbackPower_Convert/1
  BMS5_FeedbackPower_Convert/1 -> BMS5_FeedbackPower_L/1
  BMS5_FeedbackPower_L/1 -> BMS5_FeedbackPower_S/1
  BMS5_FeedbackPower_S/1 -> BMS5_FeedbackPowercv/1
  BMS5_FeedbackPowercv/1 -> BMS5_FeedbackPower_F/1
  BMS5_FailureLevel_F/1 -> BMS5_FailureLevel_Ad/1
  BMS5_FailureLevel_O/1 -> BMS5_FailureLevel_Ad/2
  BMS5_FailureLevel_Ad/1 -> BMS5_FailureLevel_sat/1
  BMS5_FailureLevel_sat/1 -> BMS5_FailureLevel_Out/1
  Demux/1 -> BMS5_FailureLevel_Sub/1(In1)
  BMS5_FailureLevel_Sub/1(Out1) -> BMS5_FailureLevel_Convert/1
  BMS5_FailureLevel_Convert/1 -> BMS5_FailureLevel_L/1
  BMS5_FailureLevel_L/1 -> BMS5_FailureLevel_S/1
  BMS5_FailureLevel_S/1 -> BMS5_FailureLevelcv/1
  BMS5_FailureLevelcv/1 -> BMS5_FailureLevel_F/1
  BMS5_ContDischargePower_F/1 -> BMS5_ContDischargePower_Ad/1
  BMS5_ContDischargePower_O/1 -> BMS5_ContDischargePower_Ad/2
  BMS5_ContDischargePower_Ad/1 -> BMS5_ContDischargePower_sat/1
  BMS5_ContDischargePower_sat/1 -> BMS5_ContDischargePower_Out/1
  Demux/2 -> BMS5_ContDischargePowerinput2_P/1
  BMS5_ContDischargePowerinput2_C/1 -> BMS5_ContDischargePowerinput2_P/2
  BMS5_ContDischargePowerinput2_P/1 -> BMS5_ContDischargePowerinput2_Ad/1
  Demux/3 -> BMS5_ContDischargePowerinput2_Ad/2
  BMS5_ContDischargePowerinput2_Ad/1 -> BMS5_ContDischargePower_Sub/1(In1)
  BMS5_ContDischargePower_Sub/1(Out1) -> BMS5_ContDischargePower_Convert/1
  BMS5_ContDischargePower_Convert/1 -> BMS5_ContDischargePower_L/1
  BMS5_ContDischargePower_L/1 -> BMS5_ContDischargePower_S/1
  BMS5_ContDischargePower_S/1 -> BMS5_ContDischargePowercv/1
  BMS5_ContDischargePowercv/1 -> BMS5_ContDischargePower_F/1
  BMS5_15s_InstanceDisPower_F/1 -> BMS5_15s_InstanceDisPower_Ad/1
  BMS5_15s_InstanceDisPower_O/1 -> BMS5_15s_InstanceDisPower_Ad/2
  BMS5_15s_InstanceDisPower_Ad/1 -> BMS5_15s_InstanceDisPower_sat/1
  BMS5_15s_InstanceDisPower_sat/1 -> BMS5_15s_InstanceDisPower_Out/1
  Demux/4 -> BMS5_15s_InstanceDisPowerinput4_P/1
  BMS5_15s_InstanceDisPowerinput4_C/1 -> BMS5_15s_InstanceDisPowerinput4_P/2
  BMS5_15s_InstanceDisPowerinput4_P/1 -> BMS5_15s_InstanceDisPowerinput4_Ad/1
  Demux/5 -> BMS5_15s_InstanceDisPowerinput4_Ad/2
  BMS5_15s_InstanceDisPowerinput4_Ad/1 -> BMS5_15s_InstanceDisPower_Sub/1(In1)
  BMS5_15s_InstanceDisPower_Sub/1(Out1) -> BMS5_15s_InstanceDisPower_Convert/1
  BMS5_15s_InstanceDisPower_Convert/1 -> BMS5_15s_InstanceDisPower_L/1
  BMS5_15s_InstanceDisPower_L/1 -> BMS5_15s_InstanceDisPower_S/1
  BMS5_15s_InstanceDisPower_S/1 -> BMS5_15s_InstanceDisPowercv/1
  BMS5_15s_InstanceDisPowercv/1 -> BMS5_15s_InstanceDisPower_F/1
  input/1 -> Demux/1

== system six_plus_six_AcmsteeringV09_main_2lflm/Data_input/Enabled Subsystem/Subsystem ==
  CANTransmit : ec5744lib/RapidECU_U3/04CANCommunication/CANTransmit  canmodule=1  canbuffer=59  canmessageid=hex2dec('0000')  canmessagetype=Standard(11-bit ID)  datalength=2  sampletime=-1
  Constant2 : Constant  Value=hex2dec('00')  SampleTime=-1
  Constant3 : Constant  Value=hex2dec('01')  SampleTime=-1
  Data Type Conversion3 : DataTypeConversion
  Data Type Conversion8 : DataTypeConversion
  Mux : Mux  Inputs=2
  Terminator2 : Terminator
  wires:
  Mux/1 -> CANTransmit/1
  Constant3/1 -> Data Type Conversion3/1
  CANTransmit/1 -> Terminator2/1
  Data Type Conversion3/1 -> Mux/1
  Data Type Conversion8/1 -> Mux/2
  Constant2/1 -> Data Type Conversion8/1

== system six_plus_six_AcmsteeringV09_main_2lflm/Data_input/MCU0/MCU0 ==
  input : Inport
  Enable : EnablePort
  Demux : Demux  Outputs=8
  MCU0_ControlMode_Ad : Sum
  MCU0_ControlMode_Convert : DataTypeConversion  OutDataTypeStr=uint32
  MCU0_ControlMode_F : Gain
  MCU0_ControlMode_L : simulink/Logic and Bit Operations/Bitwise Operator  logicop=AND  UseBitMask=on  BitMask=4  BitMaskRealWorld=Stored Integer
  MCU0_ControlMode_O : Constant  Value=0  OutDataTypeStr=single
  MCU0_ControlMode_S : ArithShift  BitShiftNumber=2
  MCU0_ControlMode_Sub : Subsystem
  MCU0_ControlMode_sat : Saturate  UpperLimit=1  LowerLimit=0
  MCU0_ControlModecv : DataTypeConversion
  MCU0_EmergShutDown_Ad : Sum
  MCU0_EmergShutDown_Convert : DataTypeConversion  OutDataTypeStr=uint32
  MCU0_EmergShutDown_F : Gain
  MCU0_EmergShutDown_L : simulink/Logic and Bit Operations/Bitwise Operator  logicop=AND  UseBitMask=on  BitMask=128  BitMaskRealWorld=Stored Integer
  MCU0_EmergShutDown_O : Constant  Value=0  OutDataTypeStr=single
  MCU0_EmergShutDown_S : ArithShift  BitShiftNumber=7
  MCU0_EmergShutDown_Sub : Subsystem
  MCU0_EmergShutDown_sat : Saturate  UpperLimit=1  LowerLimit=0
  MCU0_EmergShutDowncv : DataTypeConversion
  MCU0_GearStatus_Ad : Sum
  MCU0_GearStatus_Convert : DataTypeConversion  OutDataTypeStr=uint32
  MCU0_GearStatus_F : Gain
  MCU0_GearStatus_L : simulink/Logic and Bit Operations/Bitwise Operator  logicop=AND  UseBitMask=on  BitMask=24  BitMaskRealWorld=Stored Integer
  MCU0_GearStatus_O : Constant  Value=0  OutDataTypeStr=single
  MCU0_GearStatus_S : ArithShift  BitShiftNumber=3
  MCU0_GearStatus_Sub : Subsystem
  MCU0_GearStatus_sat : Saturate  UpperLimit=3  LowerLimit=0
  MCU0_GearStatuscv : DataTypeConversion
  MCU0_HighVol_Ad : Sum
  MCU0_HighVol_Convert : DataTypeConversion  OutDataTypeStr=uint32
  MCU0_HighVol_F : Gain
  MCU0_HighVol_L : simulink/Logic and Bit Operations/Bitwise Operator  logicop=AND  UseBitMask=on  BitMask=32  BitMaskRealWorld=Stored Integer
  MCU0_HighVol_O : Constant  Value=0  OutDataTypeStr=single
  MCU0_HighVol_S : ArithShift  BitShiftNumber=5
  MCU0_HighVol_Sub : Subsystem
  MCU0_HighVol_sat : Saturate  UpperLimit=1  LowerLimit=0
  MCU0_HighVolcv : DataTypeConversion
  MCU0_LiftCnt_Ad : Sum
  MCU0_LiftCnt_Convert : DataTypeConversion  OutDataTypeStr=uint32
  MCU0_LiftCnt_F : Gain
  MCU0_LiftCnt_L : simulink/Logic and Bit Operations/Bitwise Operator  logicop=AND  UseBitMask=on  BitMask=255  BitMaskRealWorld=Stored Integer
  MCU0_LiftCnt_O : Constant  Value=0  OutDataTypeStr=single
  MCU0_LiftCnt_S : ArithShift
  MCU0_LiftCnt_Sub : Subsystem
  MCU0_LiftCnt_sat : Saturate  UpperLimit=255  LowerLimit=0
  MCU0_LiftCntcv : DataTypeConversion
  MCU0_ShutDowAllow_Ad : Sum
  MCU0_ShutDowAllow_Convert : DataTypeConversion  OutDataTypeStr=uint32
  MCU0_ShutDowAllow_F : Gain
  MCU0_ShutDowAllow_L : simulink/Logic and Bit Operations/Bitwise Operator  logicop=AND  UseBitMask=on  BitMask=64  BitMaskRealWorld=Stored Integer
  MCU0_ShutDowAllow_O : Constant  Value=0  OutDataTypeStr=single
  MCU0_ShutDowAllow_S : ArithShift  BitShiftNumber=6
  MCU0_ShutDowAllow_Sub : Subsystem
  MCU0_ShutDowAllow_sat : Saturate  UpperLimit=1  LowerLimit=0
  MCU0_ShutDowAllowcv : DataTypeConversion
  MCU0_SpeedFdk_Ad : Sum
  MCU0_SpeedFdk_Convert : DataTypeConversion  OutDataTypeStr=uint32
  MCU0_SpeedFdk_F : Gain
  MCU0_SpeedFdk_L : simulink/Logic and Bit Operations/Bitwise Operator  logicop=AND  UseBitMask=on  BitMask=65535  BitMaskRealWorld=Stored Integer
  MCU0_SpeedFdk_O : Constant  Value=-10000  OutDataTypeStr=single
  MCU0_SpeedFdk_S : ArithShift
  MCU0_SpeedFdk_Sub : Subsystem
  MCU0_SpeedFdk_sat : Saturate  UpperLimit=10000  LowerLimit=-10000
  MCU0_SpeedFdkcv : DataTypeConversion
  MCU0_SpeedFdkinput2_Ad : Sum
  MCU0_SpeedFdkinput2_C : Constant  Value=256
  MCU0_SpeedFdkinput2_P : Product
  MCU0_TorqueFdk_Ad : Sum
  MCU0_TorqueFdk_Convert : DataTypeConversion  OutDataTypeStr=uint32
  MCU0_TorqueFdk_F : Gain  Gain=0.1
  MCU0_TorqueFdk_L : simulink/Logic and Bit Operations/Bitwise Operator  logicop=AND  UseBitMask=on  BitMask=65535  BitMaskRealWorld=Stored Integer
  MCU0_TorqueFdk_O : Constant  Value=-1000  OutDataTypeStr=single
  MCU0_TorqueFdk_S : ArithShift
  MCU0_TorqueFdk_Sub : Subsystem
  MCU0_TorqueFdk_sat : Saturate  UpperLimit=1000  LowerLimit=-1000
  MCU0_TorqueFdkcv : DataTypeConversion
  MCU0_TorqueFdkinput4_Ad : Sum
  MCU0_TorqueFdkinput4_C : Constant  Value=256
  MCU0_TorqueFdkinput4_P : Product
  MCU0_TorqueMax_Ad : Sum
  MCU0_TorqueMax_Convert : DataTypeConversion  OutDataTypeStr=uint32
  MCU0_TorqueMax_F : Gain  Gain=0.1
  MCU0_TorqueMax_L : simulink/Logic and Bit Operations/Bitwise Operator  logicop=AND  UseBitMask=on  BitMask=65535  BitMaskRealWorld=Stored Integer
  MCU0_TorqueMax_O : Constant  Value=-1000  OutDataTypeStr=single
  MCU0_TorqueMax_S : ArithShift
  MCU0_TorqueMax_Sub : Subsystem
  MCU0_TorqueMax_sat : Saturate  UpperLimit=1000  LowerLimit=-1000
  MCU0_TorqueMaxcv : DataTypeConversion
  MCU0_TorqueMaxinput6_Ad : Sum
  MCU0_TorqueMaxinput6_C : Constant  Value=256
  MCU0_TorqueMaxinput6_P : Product
  MCU0_WorkStatus_Ad : Sum
  MCU0_WorkStatus_Convert : DataTypeConversion  OutDataTypeStr=uint32
  MCU0_WorkStatus_F : Gain
  MCU0_WorkStatus_L : simulink/Logic and Bit Operations/Bitwise Operator  logicop=AND  UseBitMask=on  BitMask=3  BitMaskRealWorld=Stored Integer
  MCU0_WorkStatus_O : Constant  Value=0  OutDataTypeStr=single
  MCU0_WorkStatus_S : ArithShift
  MCU0_WorkStatus_Sub : Subsystem
  MCU0_WorkStatus_sat : Saturate  UpperLimit=3  LowerLimit=0
  MCU0_WorkStatuscv : DataTypeConversion
  MCU0_TorqueMax_Out : Outport
  MCU0_EmergShutDown_Out : Outport  Port=2
  MCU0_ShutDowAllow_Out : Outport  Port=3
  MCU0_HighVol_Out : Outport  Port=4
  MCU0_LiftCnt_Out : Outport  Port=5
  MCU0_TorqueFdk_Out : Outport  Port=6
  MCU0_SpeedFdk_Out : Outport  Port=7
  MCU0_GearStatus_Out : Outport  Port=8
  MCU0_ControlMode_Out : Outport  Port=9
  MCU0_WorkStatus_Out : Outport  Port=10
  wires:
  MCU0_TorqueMax_F/1 -> MCU0_TorqueMax_Ad/1
  MCU0_TorqueMax_O/1 -> MCU0_TorqueMax_Ad/2
  MCU0_TorqueMax_Ad/1 -> MCU0_TorqueMax_sat/1
  MCU0_TorqueMax_sat/1 -> MCU0_TorqueMax_Out/1
  Demux/6 -> MCU0_TorqueMaxinput6_P/1
  MCU0_TorqueMaxinput6_C/1 -> MCU0_TorqueMaxinput6_P/2
  MCU0_TorqueMaxinput6_P/1 -> MCU0_TorqueMaxinput6_Ad/1
  Demux/7 -> MCU0_TorqueMaxinput6_Ad/2
  MCU0_TorqueMaxinput6_Ad/1 -> MCU0_TorqueMax_Sub/1(In1)
  MCU0_TorqueMax_Sub/1(Out1) -> MCU0_TorqueMax_Convert/1
  MCU0_TorqueMax_Convert/1 -> MCU0_TorqueMax_L/1
  MCU0_TorqueMax_L/1 -> MCU0_TorqueMax_S/1
  MCU0_TorqueMax_S/1 -> MCU0_TorqueMaxcv/1
  MCU0_TorqueMaxcv/1 -> MCU0_TorqueMax_F/1
  MCU0_EmergShutDown_F/1 -> MCU0_EmergShutDown_Ad/1
  MCU0_EmergShutDown_O/1 -> MCU0_EmergShutDown_Ad/2
  MCU0_EmergShutDown_Ad/1 -> MCU0_EmergShutDown_sat/1
  MCU0_EmergShutDown_sat/1 -> MCU0_EmergShutDown_Out/1
  Demux/1 -> MCU0_ControlMode_Sub/1(In1), MCU0_WorkStatus_Sub/1(In1), MCU0_GearStatus_Sub/1(In1), MCU0_HighVol_Sub/1(In1), MCU0_ShutDowAllow_Sub/1(In1), MCU0_EmergShutDown_Sub/1(In1)
  MCU0_EmergShutDown_Sub/1(Out1) -> MCU0_EmergShutDown_Convert/1
  MCU0_EmergShutDown_Convert/1 -> MCU0_EmergShutDown_L/1
  MCU0_EmergShutDown_L/1 -> MCU0_EmergShutDown_S/1
  MCU0_EmergShutDown_S/1 -> MCU0_EmergShutDowncv/1
  MCU0_EmergShutDowncv/1 -> MCU0_EmergShutDown_F/1
  MCU0_ShutDowAllow_F/1 -> MCU0_ShutDowAllow_Ad/1
  MCU0_ShutDowAllow_O/1 -> MCU0_ShutDowAllow_Ad/2
  MCU0_ShutDowAllow_Ad/1 -> MCU0_ShutDowAllow_sat/1
  MCU0_ShutDowAllow_sat/1 -> MCU0_ShutDowAllow_Out/1
  MCU0_ShutDowAllow_Sub/1(Out1) -> MCU0_ShutDowAllow_Convert/1
  MCU0_ShutDowAllow_Convert/1 -> MCU0_ShutDowAllow_L/1
  MCU0_ShutDowAllow_L/1 -> MCU0_ShutDowAllow_S/1
  MCU0_ShutDowAllow_S/1 -> MCU0_ShutDowAllowcv/1
  MCU0_ShutDowAllowcv/1 -> MCU0_ShutDowAllow_F/1
  MCU0_HighVol_F/1 -> MCU0_HighVol_Ad/1
  MCU0_HighVol_O/1 -> MCU0_HighVol_Ad/2
  MCU0_HighVol_Ad/1 -> MCU0_HighVol_sat/1
  MCU0_HighVol_sat/1 -> MCU0_HighVol_Out/1
  MCU0_HighVol_Sub/1(Out1) -> MCU0_HighVol_Convert/1
  MCU0_HighVol_Convert/1 -> MCU0_HighVol_L/1
  MCU0_HighVol_L/1 -> MCU0_HighVol_S/1
  MCU0_HighVol_S/1 -> MCU0_HighVolcv/1
  MCU0_HighVolcv/1 -> MCU0_HighVol_F/1
  MCU0_LiftCnt_F/1 -> MCU0_LiftCnt_Ad/1
  MCU0_LiftCnt_O/1 -> MCU0_LiftCnt_Ad/2
  MCU0_LiftCnt_Ad/1 -> MCU0_LiftCnt_sat/1
  MCU0_LiftCnt_sat/1 -> MCU0_LiftCnt_Out/1
  Demux/8 -> MCU0_LiftCnt_Sub/1(In1)
  MCU0_LiftCnt_Sub/1(Out1) -> MCU0_LiftCnt_Convert/1
  MCU0_LiftCnt_Convert/1 -> MCU0_LiftCnt_L/1
  MCU0_LiftCnt_L/1 -> MCU0_LiftCnt_S/1
  MCU0_LiftCnt_S/1 -> MCU0_LiftCntcv/1
  MCU0_LiftCntcv/1 -> MCU0_LiftCnt_F/1
  MCU0_TorqueFdk_F/1 -> MCU0_TorqueFdk_Ad/1
  MCU0_TorqueFdk_O/1 -> MCU0_TorqueFdk_Ad/2
  MCU0_TorqueFdk_Ad/1 -> MCU0_TorqueFdk_sat/1
  MCU0_TorqueFdk_sat/1 -> MCU0_TorqueFdk_Out/1
  Demux/4 -> MCU0_TorqueFdkinput4_P/1
  MCU0_TorqueFdkinput4_C/1 -> MCU0_TorqueFdkinput4_P/2
  MCU0_TorqueFdkinput4_P/1 -> MCU0_TorqueFdkinput4_Ad/1
  Demux/5 -> MCU0_TorqueFdkinput4_Ad/2
  MCU0_TorqueFdkinput4_Ad/1 -> MCU0_TorqueFdk_Sub/1(In1)
  MCU0_TorqueFdk_Sub/1(Out1) -> MCU0_TorqueFdk_Convert/1
  MCU0_TorqueFdk_Convert/1 -> MCU0_TorqueFdk_L/1
  MCU0_TorqueFdk_L/1 -> MCU0_TorqueFdk_S/1
  MCU0_TorqueFdk_S/1 -> MCU0_TorqueFdkcv/1
  MCU0_TorqueFdkcv/1 -> MCU0_TorqueFdk_F/1
  MCU0_SpeedFdk_F/1 -> MCU0_SpeedFdk_Ad/1
  MCU0_SpeedFdk_O/1 -> MCU0_SpeedFdk_Ad/2
  MCU0_SpeedFdk_Ad/1 -> MCU0_SpeedFdk_sat/1
  MCU0_SpeedFdk_sat/1 -> MCU0_SpeedFdk_Out/1
  Demux/2 -> MCU0_SpeedFdkinput2_P/1
  MCU0_SpeedFdkinput2_C/1 -> MCU0_SpeedFdkinput2_P/2
  MCU0_SpeedFdkinput2_P/1 -> MCU0_SpeedFdkinput2_Ad/1
  Demux/3 -> MCU0_SpeedFdkinput2_Ad/2
  MCU0_SpeedFdkinput2_Ad/1 -> MCU0_SpeedFdk_Sub/1(In1)
  MCU0_SpeedFdk_Sub/1(Out1) -> MCU0_SpeedFdk_Convert/1
  MCU0_SpeedFdk_Convert/1 -> MCU0_SpeedFdk_L/1
  MCU0_SpeedFdk_L/1 -> MCU0_SpeedFdk_S/1
  MCU0_SpeedFdk_S/1 -> MCU0_SpeedFdkcv/1
  MCU0_SpeedFdkcv/1 -> MCU0_SpeedFdk_F/1
  MCU0_GearStatus_F/1 -> MCU0_GearStatus_Ad/1
  MCU0_GearStatus_O/1 -> MCU0_GearStatus_Ad/2
  MCU0_GearStatus_Ad/1 -> MCU0_GearStatus_sat/1
  MCU0_GearStatus_sat/1 -> MCU0_GearStatus_Out/1
  MCU0_GearStatus_Sub/1(Out1) -> MCU0_GearStatus_Convert/1
  MCU0_GearStatus_Convert/1 -> MCU0_GearStatus_L/1
  MCU0_GearStatus_L/1 -> MCU0_GearStatus_S/1
  MCU0_GearStatus_S/1 -> MCU0_GearStatuscv/1
  MCU0_GearStatuscv/1 -> MCU0_GearStatus_F/1
  MCU0_ControlMode_F/1 -> MCU0_ControlMode_Ad/1
  MCU0_ControlMode_O/1 -> MCU0_ControlMode_Ad/2
  MCU0_ControlMode_Ad/1 -> MCU0_ControlMode_sat/1
  MCU0_ControlMode_sat/1 -> MCU0_ControlMode_Out/1
  MCU0_ControlMode_Sub/1(Out1) -> MCU0_ControlMode_Convert/1
  MCU0_ControlMode_Convert/1 -> MCU0_ControlMode_L/1
  MCU0_ControlMode_L/1 -> MCU0_ControlMode_S/1
  MCU0_ControlMode_S/1 -> MCU0_ControlModecv/1
  MCU0_ControlModecv/1 -> MCU0_ControlMode_F/1
  MCU0_WorkStatus_F/1 -> MCU0_WorkStatus_Ad/1
  MCU0_WorkStatus_O/1 -> MCU0_WorkStatus_Ad/2
  MCU0_WorkStatus_Ad/1 -> MCU0_WorkStatus_sat/1
  MCU0_WorkStatus_sat/1 -> MCU0_WorkStatus_Out/1
  MCU0_WorkStatus_Sub/1(Out1) -> MCU0_WorkStatus_Convert/1
  MCU0_WorkStatus_Convert/1 -> MCU0_WorkStatus_L/1
  MCU0_WorkStatus_L/1 -> MCU0_WorkStatus_S/1
  MCU0_WorkStatus_S/1 -> MCU0_WorkStatuscv/1
  MCU0_WorkStatuscv/1 -> MCU0_WorkStatus_F/1
  input/1 -> Demux/1

== matlab function six_plus_six_AcmsteeringV09_main_2lflm/MainControl/mode_control/forward/forward/Drive/左右侧电机分配及功率限制/MATLAB Function ==
  data: trqlim_l input; trq_dem_l output; trq_dem_r output; trq_dem_l1 input; trqlim_r input; trq_dem_r1 input; delta_T_dem input
function [trq_dem_l,trq_dem_r] = fcn(trqlim_l,trq_dem_l1,trqlim_r,trq_dem_r1,delta_T_dem)
%#codegen
if trq_dem_l1==trqlim_l
    trq_dem_l=single(trq_dem_l1);
    trq_dem_r=single(trq_dem_l1+delta_T_dem);%这时候加的是负值
elseif trq_dem_r1==trqlim_r
    trq_dem_l=single(trq_dem_r1-delta_T_dem);
    trq_dem_r=single(trq_dem_r1);
    
else
    trq_dem_l=single(trq_dem_l1);
    trq_dem_r=single(trq_dem_r1);
end
% trq_dem_l=single(max(0,trq_dem_l));%限一下最小值，不要小于0
% trq_dem_r=single(max(0,trq_dem_r));
trq_dem_l=single(max(-trqlim_l,trq_dem_l));%小转向半径下，内侧履带是可能输出负转矩的，从地面吸收功率，给外侧，所以不能限到0，限到最大电机外特性负值
trq_dem_r=single(max(-trqlim_r,trq_dem_r));
end

== matlab function six_plus_six_AcmsteeringV09_main_2lflm/MainControl/mode_control/forward/forward/Drive/驱动防滑控制TCS/直行TCS/直行/HeartBeat3 ==
  data: life_pre input; life output
function life = fcn(life_pre)
%#codegen
life=single(life_pre+1);
if life>255
    life=single(0);
end
end

== matlab function six_plus_six_AcmsteeringV09_main_2lflm/MainControl/mode_control/forward/forward/Drive/驱动防滑控制TCS/直行TCS/直行/HeartBeat4 ==
  data: life_pre input; life output
function life = fcn(life_pre)
%#codegen
life=single(life_pre+1);
if life>255
    life=single(0);
end
end

== matlab function six_plus_six_AcmsteeringV09_main_2lflm/MainControl/mode_control/forward/forward/Drive/驱动防滑控制TCS/直行TCS/直行/HeartBeat1 ==
  data: life_pre input; life output
function life = fcn(life_pre)
%#codegen
life=single(life_pre+1);
if life>255
    life=single(0);
end
end

== matlab function six_plus_six_AcmsteeringV09_main_2lflm/MainControl/mode_control/forward/forward/Drive/驱动防滑控制TCS/直行TCS/直行/HeartBeat5 ==
  data: life_pre input; life output
function life = fcn(life_pre)
%#codegen
life=single(life_pre+1);
if life>255
    life=single(0);
end
end

== matlab function six_plus_six_AcmsteeringV09_main_2lflm/MainControl/mode_control/forward/forward/Brake/HeartBeat2 ==
  data: life_pre input; life output
function life = fcn(life_pre)
%#codegen
life=single(life_pre+1);
if life>255
    life=single(0);
end
end

== matlab function six_plus_six_AcmsteeringV09_main_2lflm/MainControl/mode_control/forward/forward/Brake/HeartBeat3 ==
  data: life_pre input; life output
function life = fcn(life_pre)
%#codegen
life=single(life_pre+1);
if life>255
    life=single(0);
end
end

== matlab function six_plus_six_AcmsteeringV09_main_2lflm/MainControl/mode_control/forward/forward/Brake/HeartBeat4 ==
  data: life_pre input; life output
function life = fcn(life_pre)
%#codegen
life=single(life_pre+1);
if life>255
    life=single(0);
end
end

== matlab function six_plus_six_AcmsteeringV09_main_2lflm/MainControl/mode_control/forward/forward/Brake/HeartBeat1 ==
  data: life_pre input; life output
function life = fcn(life_pre)
%#codegen
life=single(life_pre+1);
if life>255
    life=single(0);
end
end

== matlab function six_plus_six_AcmsteeringV09_main_2lflm/MainControl/mode_control/forward/forward/Brake/HeartBeat5 ==
  data: life_pre input; life output
function life = fcn(life_pre)
%#codegen
life=single(life_pre+1);
if life>255
    life=single(0);
end
end

== matlab function six_plus_six_AcmsteeringV09_main_2lflm/Data_input/3/Enabled Subsystem/MATLAB Function1 ==
  data: current_in input; current_out output
function current_out = motec_current(current_in)
    if current_in>32768
        current_out=current_in-65535;
    else
        current_out=current_in;
    end
end

== matlab function six_plus_six_AcmsteeringV09_main_2lflm/Data_input/3/Enabled Subsystem/MATLAB Function3 ==
  data: speed input; speed_out output
function speed_out = motec_speed(speed)
    if speed>32768
        speed_out=speed-65535;
    else speed_out=speed;
    end
end

== matlab function six_plus_six_AcmsteeringV09_main_2lflm/MainControl/mode_control/neutral/neutral/HeartBeat3 ==
  data: life_pre input; life output
function life = fcn(life_pre)
%#codegen
life=single(life_pre+1);
if life>255
    life=single(0);
end
end

== matlab function six_plus_six_AcmsteeringV09_main_2lflm/MainControl/mode_control/backward/backward/Brake/HeartBeat1 ==
  data: life_pre input; life output
function life = fcn(life_pre)
%#codegen
life=single(life_pre+1);
if life>255
    life=single(0);
end
end

== matlab function six_plus_six_AcmsteeringV09_main_2lflm/MainControl/mode_control/backward/backward/Brake/HeartBeat3 ==
  data: life_pre input; life output
function life = fcn(life_pre)
%#codegen
life=single(life_pre+1);
if life>255
    life=single(0);
end
end

== matlab function six_plus_six_AcmsteeringV09_main_2lflm/MainControl/mode_control/backward/backward/Brake/HeartBeat5 ==
  data: life_pre input; life output
function life = fcn(life_pre)
%#codegen
life=single(life_pre+1);
if life>255
    life=single(0);
end
end
